simulink model "zad_no_2"  (R2017b)
settings: Solver=VariableStepAuto  StartTime=0.0  StopTime=40  RelTol=1e-3
undefined symbols (not defined in the file): den, Ini, num, Tp
settings Model: Creator=micha  LastModifiedBy=micha

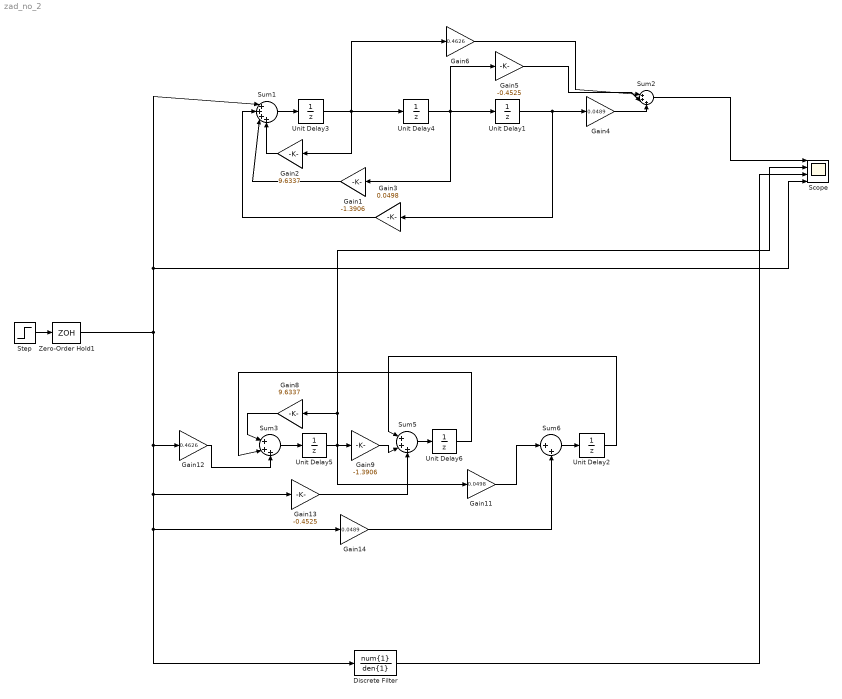
== system zad_no_2 ==
  Discrete Filter : DiscreteFilter  Numerator=num{1}  Denominator=den{1}
  Gain1 : Gain  Gain=-1.3906  ParamDataTypeStr=double
  Gain11 : Gain  Gain=0.0498  ParamDataTypeStr=double
  Gain12 : Gain  Gain=0.4626  ParamDataTypeStr=double
  Gain13 : Gain  Gain=-0.4525  ParamDataTypeStr=double
  Gain14 : Gain  Gain=0.0489  ParamDataTypeStr=double
  Gain2 : Gain  Gain=9.6337  ParamDataTypeStr=double
  Gain3 : Gain  Gain=0.0498  ParamDataTypeStr=double
  Gain4 : Gain  Gain=0.0489  ParamDataTypeStr=double
  Gain5 : Gain  Gain=-0.4525  ParamDataTypeStr=double
  Gain6 : Gain  Gain=0.4626  ParamDataTypeStr=double
  Gain8 : Gain  Gain=9.6337  ParamDataTypeStr=double
  Gain9 : Gain  Gain=-1.3906  ParamDataTypeStr=double
  Scope : Scope  NumInputPorts=4
  Step : Step  SampleTime=0
  Sum1 : Sum  Inputs=|++++
  Sum2 : Sum  Inputs=|+++
  Sum3 : Sum  Inputs=|+++
  Sum5 : Sum  Inputs=|+++
  Sum6 : Sum  Inputs=|++
  Unit Delay{1..6} (6 alike) : UnitDelay  InitialCondition=Ini  SampleTime=Tp
  Zero-Order Hold1 : ZeroOrderHold  SampleTime=Tp
  wires:
  Sum1/1 -> Unit Delay3/1
  Gain2/1 -> Sum1/4
  Unit Delay3/1 -> Gain6/1, Unit Delay4/1, Gain2/1
  Unit Delay4/1 -> Gain5/1, Gain1/1, Unit Delay1/1
  Unit Delay1/1 -> Gain4/1, Gain3/1
  Sum2/1 -> Scope/1
  Gain1/1 -> Sum1/3
  Gain3/1 -> Sum1/2
  Gain4/1 -> Sum2/3
  Gain5/1 -> Sum2/2
  Gain6/1 -> Sum2/1
  Step/1 -> Zero-Order Hold1/1
  Sum3/1 -> Unit Delay5/1
  Unit Delay2/1 -> Sum5/1
  Unit Delay6/1 -> Sum3/2
  Gain8/1 -> Sum3/1
  Sum5/1 -> Unit Delay6/1
  Gain9/1 -> Sum5/2
  Sum6/1 -> Unit Delay2/1
  Gain11/1 -> Sum6/1
  Gain12/1 -> Sum3/3
  Gain13/1 -> Sum5/3
  Gain14/1 -> Sum6/2
  Unit Delay5/1 -> Gain11/1, Scope/2, Gain8/1, Gain9/1
  Zero-Order Hold1/1 -> Gain13/1, Discrete Filter/1, Gain14/1, Gain12/1, Scope/4, Sum1/1
  Discrete Filter/1 -> Scope/3
